simulink model "PT2_regelstrecke"  (Simulink 7.6)
settings: Solver=ode45  StartTime=0.0  StopTime=0.01  RelTol=1e-3
libraries: simulink x1
settings Model: Creator=localadmin  LastModifiedBy=localadmin

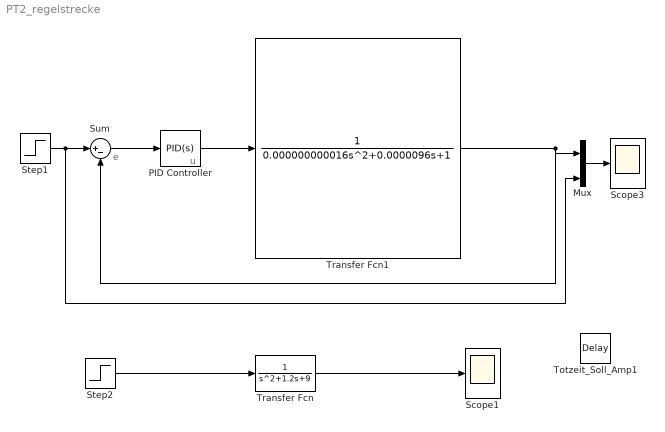
== system PT2_regelstrecke ==
  note: e
  note: u
  Mux : Mux  Inputs=2
  PID Controller : simulink/Continuous/PID Controller  DialogController=pidpack.PIDConfig.pidDDGCreate  DialogControllerArgs=DataTag0  SystemSampleTime=-1  Controller=PID  TimeDomain=Continuous-time  SampleTime=1  IntegratorMethod=Forward Euler  FilterMethod=Forward Euler  Form=Parallel  P=1  I=1000000  D=0.05  N=100  InitialConditionSource=internal  InitialConditionForIntegrator=0  InitialConditionForFilter=0  ExternalReset=none  LimitOutput=off  UpperSaturationLimit=inf  LowerSaturationLimit=-inf  LinearizeAsGain=off  AntiWindupMode=none  Kb=1  TrackingMode=off  Kt=1  PParamMin=[]  PParamMax=[]  IParamMin=[]  IParamMax=[]  DParamMin=[]  DParamMax=[]  NParamMin=[]  NParamMax=[]  KbParamMin=[]  KbParamMax=[]  KtParamMin=[]  KtParamMax=[]  POutMin=[]  POutMax=[]  IOutMin=[]  IOutMax=[]  DOutMin=[]  DOutMax=[]  NOutMin=[]  NOutMax=[]  KbOutMin=[]  KbOutMax=[]  KtOutMin=[]  KtOutMax=[]  IntegratorOutMin=[]  IntegratorOutMax=[]  FilterOutMin=[]  FilterOutMax=[]  SumOutMin=[]  SumOutMax=[]  SumI1OutMin=[]  SumI1OutMax=[]  SumI2OutMin=[]  SumI2OutMax=[]  SumI3OutMin=[]  SumI3OutMax=[]  SumDOutMin=[]  SumDOutMax=[]  SaturationOutMin=[]  SaturationOutMax=[]  IntegratorContinuousStateAttributes=''  IntegratorStateMustResolveToSignalObject=off  IntegratorRTWStateStorageClass=Auto  FilterContinuousStateAttributes=''  FilterStateMustResolveToSignalObject=off  FilterRTWStateStorageClass=Auto
  Scope1 : Scope
      settings: YMin=0.205  YMax=0.2525
  Scope3 : Scope
      settings: YMin=0.9300000000000001  YMax=1.07
  Step1 : Step  Time=0.0001  Before=1  SampleTime=1
  Step2 : Step  Time=0.0001  After=2  SampleTime=1
  Sum : Sum  Inputs=|+-  SampleTime=0
  Totzeit_Soll_Amp1 : TransportDelay  DelayTime=0.5*10^(-5)
  Transfer Fcn : TransferFcn  Denominator=[1 1.2 9]
  Transfer Fcn1 : TransferFcn  Denominator=[0.000000000016 0.0000096 1]
  wires:
  Step1/1 -> Sum/1, Mux/2
  Sum/1 -> PID Controller/1
  Mux/1 -> Scope3/1
  Transfer Fcn/1 -> Scope1/1
  PID Controller/1 -> Transfer Fcn1/1
  Transfer Fcn1/1 -> Sum/2, Mux/1
  Step2/1 -> Transfer Fcn/1
